simulink model "C_transition"  (R2020a)
settings: Solver=FixedStepDiscrete  StartTime=0.0  StopTime=200  FixedStep=0.1  RelTol=1e-3  EnableMultiTasking=on
settings Model: Creator=hp-pc  LastModifiedBy=hp-pc
settings SolverCC: AutoInsertRateTranBlk=on
settings OptimizationCC: LifeSpan=inf
settings DebuggingCC: SFUnexpectedBacktrackingDiag=warning  SFNoUnconditionalDefaultTransitionDiag=warning  SFExecutionAtInitializationDiag=none  ArithmeticOperatorsInVariantConditions=warning
settings SFSimCC: SimUseLocalCustomCode=off  CustomCodeUndefinedFunction=UseInterfaceOnly
settings RTWCC: RTWUseLocalCustomCode=off
settings CodeAppCC: StateflowObjectComments=on
settings GRTTargetCC: TargetLangStandard=C89/C90 (ANSI)
settings ConfigComp: CovMetricSettings=dw  CovHtmlReporting=on  CovSaveCumulativeToWorkspaceVar=on  CovSaveSingleToWorkspaceVar=on  CovShowResultsExplorer=off  CovExternalEMLEnable=off

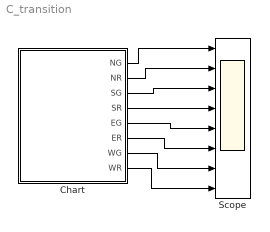
== system C_transition ==
  Chart : Stateflow chart  TreatAsAtomicUnit=on
  Scope : Scope  NumInputPorts=8
  wires:
  Chart/1(NG) -> Scope/1
  Chart/2(NR) -> Scope/2
  Chart/3(SG) -> Scope/3
  Chart/4(SR) -> Scope/4
  Chart/5(EG) -> Scope/5
  Chart/6(ER) -> Scope/6
  Chart/7(WG) -> Scope/7
  Chart/8(WR) -> Scope/8

== stateflow chart C_transition/Chart ==
  state C1
    state NB [parallel]
      NG=1;
      NR=0;
      settings: executionOrder=1
    state SB [parallel]
      SG=1;
      SR=0;
      settings: executionOrder=2
    state EB [parallel]
      EG=0;
      ER=1;
      settings: executionOrder=3
    state WB [parallel]
      WG=0;
      WR=1;
      settings: executionOrder=4
  state C2
    state NB [parallel]
      NG=0;
      NR=1;
      settings: executionOrder=1
    state SB [parallel]
      SG=0;
      SR=1;
      settings: executionOrder=2
    state EB [parallel]
      EG=1;
      ER=0;
      settings: executionOrder=3
    state WB [parallel]
      WG=1;
      WR=0;
      settings: executionOrder=4
  (default) -> C1
  C1 -> C2 : after(90,sec)
  C2 -> C1 : after(90,sec)
  data: NG output; NR output; SG output; SR output; EG output; ER output; WG output; WR output
